simulink model "projectURJA"  (R2023b)
settings: Solver=VariableStepAuto  StartTime=0.0  StopTime=2  MaxStep=1e-4  RelTol=1e-3
libraries: spsCurrentMeasurementLib x2, spsGroundLib x2, spsVoltageMeasurementLib x2, spsDCMachineLib x1, spsDCVoltageSourceLib x1, spsPVArrayLib x1, spsSeriesRLCBranchLib x1, spsWindTurbineLib x1, sps_lib x1
settings Model: Creator=HP  LastModifiedBy=Shamiul
settings SolverCC: AlgebraicLoopSolver=TrustRegion
settings DataIOCC: ReturnWorkspaceOutputs=off
settings DebuggingCC: UnconnectedInputMsg=warning  UnconnectedOutputMsg=warning  UnconnectedLineMsg=warning  ArithmeticOperatorsInVariantConditions=warning
settings ModelReferenceCC: EnableRefExpFcnMdlSchedulingChecks=on
settings SFSimCC: SimUseLocalCustomCode=off  CustomCodeUndefinedFunction=UseInterfaceOnly
settings RTWCC: RTWUseLocalCustomCode=off
settings CodeAppCC: StateflowObjectComments=on
settings SimscapeCC: SimscapeNormalizeSystem=off

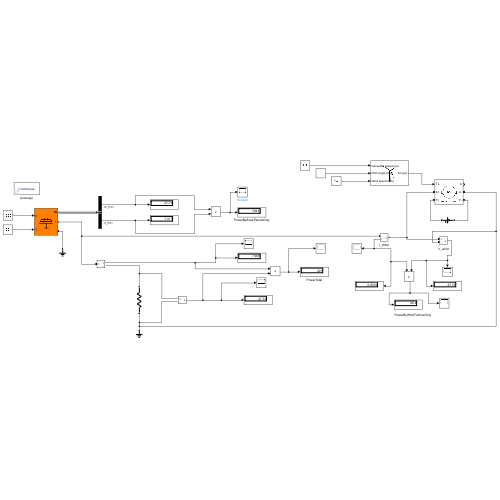
[thumbnail: Simulink's stored preview of the top-level diagram]
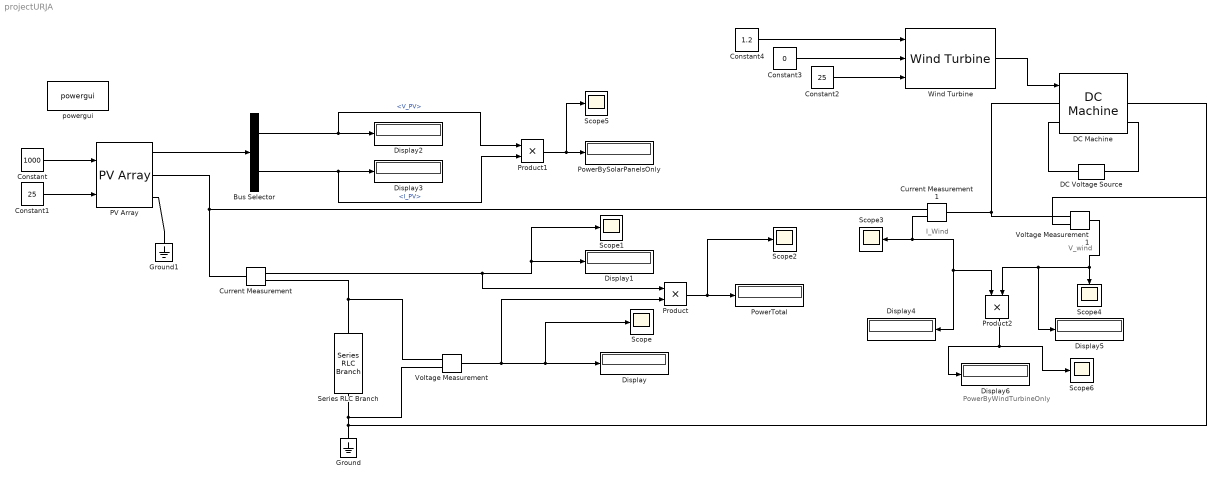
== system projectURJA ==
  note: PowerByWindTurbineOnly
  note: V_wind
  note: I_Wind
  Bus Selector : BusSelector  OutputSignals=V_PV,I_PV
  Constant : Constant  Value=1000
  Constant1 : Constant  Value=25
  Constant2 : Constant  Value=25
  Constant3 : Constant  Value=0
  Constant4 : Constant  Value=1.2
  Current Measurement : spsCurrentMeasurementLib/Current Measurement  PhasorSimulation=off  OutputType=Complex  PSBequivalent=0
  Current Measurement1 : spsCurrentMeasurementLib/Current Measurement  PhasorSimulation=off  OutputType=Complex  PSBequivalent=0
  DC Machine : spsDCMachineLib/DC Machine  PresetModel=01: 5HP 240V 1750RPM Field:300V  MechanicalLoad=Torque TL  FieldType=Wound  ShowDetailedParameters=on  MeasurementBus=off  RLa=[2.581 0.028]  RLf=[281.2 156]  Laf=0.9483  MachineConstant=Torque constant (N.m/A)  Ke=1.8  Kt=1.8  J=0.02215  Bm=0.002953  Tf=0.5161  w0=1  Ifinit=0.355618776671408  TsPowergui=0  TsBlock=-1
  DC Voltage Source : spsDCVoltageSourceLib/DC Voltage Source  Amplitude=100  Measurements=None
  Display{,1..6} (7 alike) : Display
  Ground : spsGroundLib/Ground  LConnTagsString=a
  Ground1 : spsGroundLib/Ground  LConnTagsString=a
  PV Array : spsPVArrayLib/PV Array  Npar=1  Nser=1  PlotType=array @ 1000 W/m2 & specified temperatures  S_vec="[ 1000  500  100 ]"  Temp_C_vec="[ 45 25  ]"  ModuleName=User-defined  PlotWhenSelected=off  Pm=200.112  Ncell=54  Voc=32.9  Isc=8.21  Vm=26.4  Im=7.58  beta_Voc_pc=-0.36099  alpha_Isc_pc=0.102  beta_Voc=-0.11877  alpha_Isc=0.0083742  IL=8.2311  I0=3.0465e-10  nI=0.98858  Rsh=126.9934  Rs=0.32653  RobustModel=off  RobustCellTemperature=313.3991  BAL=off  Tc=1e-6  Tfilter=5e-5
  PowerBySolarPanelsOnly : Display
  PowerTotal : Display
  Product : Product
  Product1 : Product
  Product2 : Product
  Scope{,1..6} (7 alike) : Scope
  Series RLC Branch : spsSeriesRLCBranchLib/Series RLC Branch  LConnTagsString=__new0  RConnTagsString=__new0  BranchType=R  Resistance=3.48  Inductance=1e-3  SetiL0=off  InitialCurrent=0  Capacitance=1e-6  Setx0=off  InitialVoltage=0  Measurements=None
  Voltage Measurement : spsVoltageMeasurementLib/Voltage Measurement  PhasorSimulation=off  OutputType=Complex  PSBequivalent=0
  Voltage Measurement1 : spsVoltageMeasurementLib/Voltage Measurement  PhasorSimulation=off  OutputType=Complex  PSBequivalent=0
  Wind Turbine : spsWindTurbineLib/Wind Turbine  Pnom=1.5e6  Pelec_base=1.5e6/0.9  wind_base=12  P_wind_base=0.73  speed_nom=1.2  pitch_angle=0  c1_c6="[0.51763          116          0.4            5           21     0.006795]"  cp_nom=0.48  lambda_nom=8.1
  powergui : sps_lib/powergui  Priority=1  SimulationMode=Continuous  SampleTime=50e-6  frequency=60  Iterations=50  frequencyindice=0  Pbase=100e6  ErrMax=1e-4  UnitsV=kV  UnitsW=MW  buscounter=0  FunctionMessages=off  echomessages=off  EnableUseOfTLC=off  CurrentSourceSwitches=off  DisableSnubberDevices=off  DisableRonSwitches=off  DisableVfSwitches=off  DisplayEquations=off  AutomaticDiscreteSolvers=off  SolverType=Tustin/Backward Euler (TBE)  Interpol=off  ExternalGateDelay=off  methode=off  Ts=100  x0status=blocks  SPID=on  SwTol=0  HookPort=off  NonlinearTolerance=1e-4  nMaxIteration=100  ContinueOnMaxIteration=off  RestoreLinks=warning  ResistiveCurrentMeasurement=off  Frange=[0:2:500]  Ylog=off  Xlog=on  ShowGrid=off  save=off  variable=ZData  structure=0  ZoomFFT=off  StartTime=0.0  cycles=1  DisplayStyle=1  fundamental=60  FreqAxis=off  MaxFrequency=1000  frequencyindicesteady=1  RmsSteady=1  display=off
  wires:
  Constant/1 -> PV Array/1
  Constant1/1 -> PV Array/2
  Voltage Measurement/1 -> Product/2, Scope/1, Display/1
  Current Measurement/1 -> Product/1, Scope1/1, Display1/1
  Product/1 -> Scope2/1, PowerTotal/1
  PV Array/1 -> Bus Selector/1
  Bus Selector/1 -> Product1/1, Display2/1  "<V_PV>"
  Bus Selector/2 -> Product1/2, Display3/1  "<I_PV>"
  Product1/1 -> Scope5/1, PowerBySolarPanelsOnly/1
  Constant2/1 -> Wind Turbine/3
  Constant3/1 -> Wind Turbine/2
  Wind Turbine/1 -> DC Machine/1
  Constant4/1 -> Wind Turbine/1
  Current Measurement1/1 -> Product2/1, Display4/1, Scope3/1
  Voltage Measurement1/1 -> Product2/2, Display5/1, Scope4/1
  Product2/1 -> Scope6/1, Display6/1
  connections:
  Ground/LConn1 -- Voltage Measurement1/LConn2 -- DC Machine/RConn1 -- Voltage Measurement/LConn2 -- Series RLC Branch/RConn1
  Ground1/LConn1 -- PV Array/RConn2
  Current Measurement/LConn1 -- PV Array/RConn1 -- Current Measurement1/RConn1
  Current Measurement/RConn1 -- Series RLC Branch/LConn1 -- Voltage Measurement/LConn1
  DC Voltage Source/LConn1 -- DC Machine/RConn2
  DC Voltage Source/RConn1 -- DC Machine/LConn2
  DC Machine/LConn1 -- Voltage Measurement1/LConn1 -- Current Measurement1/LConn1
